simulink model "L7task2"  (R2020a)
settings: Solver=VariableStepAuto  StartTime=0.0  StopTime=10.0  RelTol=1e-3
undefined symbols (not defined in the file): b, J, K, L, R
settings Model: Creator=bztig  LastModifiedBy=bztig

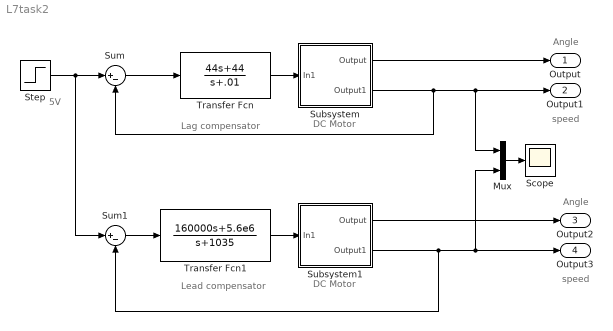
== system L7task2 ==
  note: speed
  note: Angle
  note: 5V
  note: Lag compensator
  note: DC Motor
  note: Lead compensator
  note: DC Motor
  note: speed
  note: Angle
  Mux : Mux  Inputs=2
  Scope : Scope
  Step : Step  After=5  SampleTime=0
  Subsystem : Subsystem
  Subsystem1 : Subsystem
  Sum : Sum  Inputs=|+-
  Sum1 : Sum  Inputs=|+-
  Transfer Fcn : TransferFcn  Numerator=[44 44]  Denominator=[1 .01]
  Transfer Fcn1 : TransferFcn  Numerator=[160000 5.6e6]  Denominator=[1 1035]
  Output : Outport
  Output1 : Outport  Port=2
  Output2 : Outport  Port=3
  Output3 : Outport  Port=4
  wires:
  Subsystem/1(Output) -> Output/1
  Subsystem/2(Output1) -> Mux/1, Output1/1, Sum/2
  Transfer Fcn/1 -> Subsystem/1(In1)
  Sum/1 -> Transfer Fcn/1
  Sum1/1 -> Transfer Fcn1/1
  Step/1 -> Sum1/1, Sum/1
  Transfer Fcn1/1 -> Subsystem1/1(In1)
  Subsystem1/1(Output) -> Output2/1
  Mux/1 -> Scope/1
  Subsystem1/2(Output1) -> Sum1/2, Mux/2, Output3/1

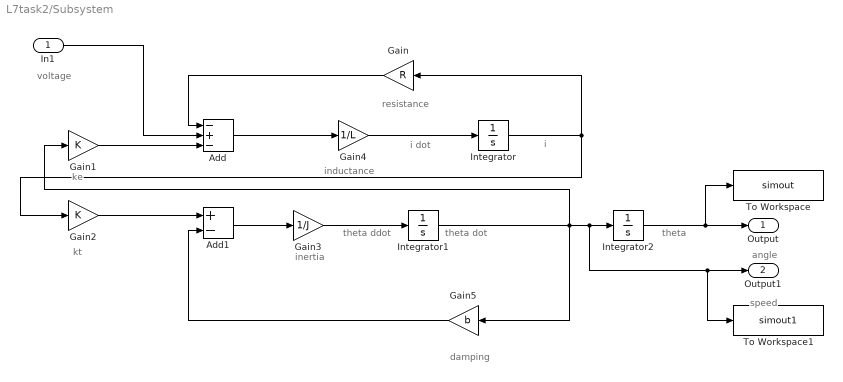
== system L7task2/Subsystem ==
  note: angle
  note: theta
  note: speed
  note: theta dot
  note: theta ddot
  note: damping
  note: resistance
  note: i
  note: i dot
  note: inertia
  note: inductance
  note: kt
  note: ke
  note: voltage
  In1 : Inport
  Add : Sum  Inputs=-+-
  Add1 : Sum  Inputs=+-
  Gain : Gain  Gain=R
  Gain1 : Gain  Gain=K
  Gain2 : Gain  Gain=K
  Gain3 : Gain  Gain=1/J
  Gain4 : Gain  Gain=1/L
  Gain5 : Gain  Gain=b
  Integrator : Integrator
  Integrator1 : Integrator
  Integrator2 : Integrator
  To Workspace : ToWorkspace  VariableName=simout  SampleTime=-1
  To Workspace1 : ToWorkspace  VariableName=simout1  SampleTime=-1
  Output : Outport
  Output1 : Outport  Port=2
  wires:
  Gain5/1 -> Add1/2
  Gain1/1 -> Add/3
  Integrator/1 -> Gain2/1, Gain/1
  Gain2/1 -> Add1/1
  Gain3/1 -> Integrator1/1
  Gain4/1 -> Integrator/1
  Add1/1 -> Gain3/1
  Add/1 -> Gain4/1
  Integrator1/1 -> Gain5/1, Gain1/1, To Workspace1/1, Output1/1, Integrator2/1
  In1/1 -> Add/2
  Integrator2/1 -> To Workspace/1, Output/1
  Gain/1 -> Add/1

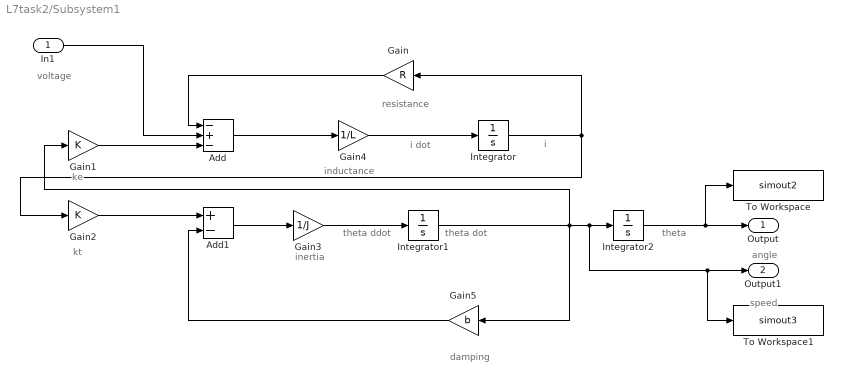
== system L7task2/Subsystem1 ==
  note: voltage
  note: ke
  note: kt
  note: inductance
  note: inertia
  note: i dot
  note: i
  note: resistance
  note: damping
  note: theta ddot
  note: theta dot
  note: speed
  note: theta
  note: angle
  In1 : Inport
  Add : Sum  Inputs=-+-
  Add1 : Sum  Inputs=+-
  Gain : Gain  Gain=R
  Gain1 : Gain  Gain=K
  Gain2 : Gain  Gain=K
  Gain3 : Gain  Gain=1/J
  Gain4 : Gain  Gain=1/L
  Gain5 : Gain  Gain=b
  Integrator : Integrator
  Integrator1 : Integrator
  Integrator2 : Integrator
  To Workspace : ToWorkspace  VariableName=simout2  SampleTime=-1
  To Workspace1 : ToWorkspace  VariableName=simout3  SampleTime=-1
  Output : Outport
  Output1 : Outport  Port=2
  wires:
  Gain/1 -> Add/1
  Integrator2/1 -> Output/1, To Workspace/1
  In1/1 -> Add/2
  Integrator1/1 -> Integrator2/1, Output1/1, To Workspace1/1, Gain1/1, Gain5/1
  Add/1 -> Gain4/1
  Add1/1 -> Gain3/1
  Gain4/1 -> Integrator/1
  Gain3/1 -> Integrator1/1
  Gain2/1 -> Add1/1
  Integrator/1 -> Gain/1, Gain2/1
  Gain1/1 -> Add/3
  Gain5/1 -> Add1/2
